simulink model "sampled_data_system"  (R2015a)
settings: Solver=ode45  StartTime=0.0  StopTime=tfinal  FixedStep=T  MaxStep=0.01  RelTol=1e-12  AbsTol=1e-12
values from neighbouring files (symbols this model uses):
  T = 0.004    [Fixed_Inner_Ctrl.mat]    (also in iop_control_design.m)
libraries: cstblocks x2
settings Model: CovHtmlReporting=off  Creator=cnielsen  LastModifiedBy=m4fisher
settings DataIOCC: LimitDataPoints=off  SignalLoggingSaveFormat=ModelDataLogs  SaveOutput=off  SaveTime=off  Refine=5
settings OptimizationCC: ExpressionDepthLimit=2147483647
settings DebuggingCC: UnderspecifiedInitializationDetection=Classic  MergeDetectMultiDrivingBlocksExec=none  SolverPrmCheckMsg=warning  FcnCallInpInsideContextMsg=EnableAllAsWarning  StateNameClashWarn=warning
settings GRTTargetCC: CombineOutputUpdateFcns=off  GRTInterface=on
settings ConfigurationSet: Description=Simscape Multibody

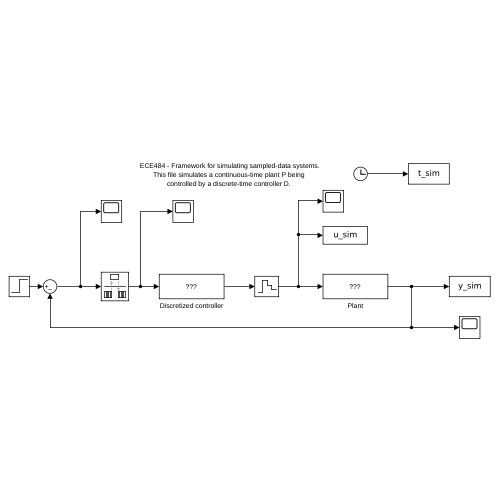
[thumbnail: Simulink's stored preview of the top-level diagram]
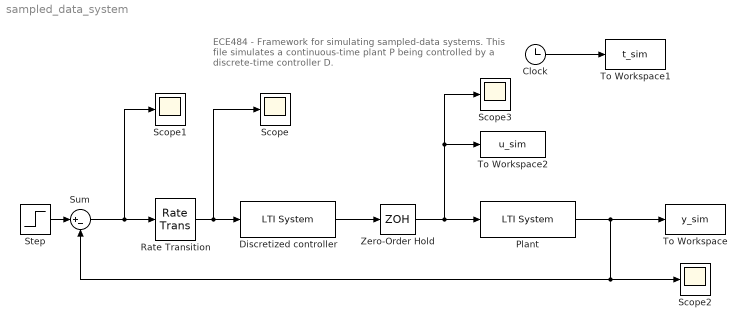
== system sampled_data_system ==
  note: ECE484 - Framework for simulating sampled-data systems.
      | This file simulates a continuous-time plant P being
      | controlled by a discrete-time controller D.
  Clock : Clock
  Discretized controller : cstblocks/LTI System  sys=D  IC=[]
  Plant : cstblocks/LTI System  sys=P  IC=[]
  Rate Transition : RateTransition  OutPortSampleTime=T
  Scope{,1..3} (4 alike) : Scope
      Scope settings: TimeRange=auto  MaxDataPoints=5000  SaveToWorkspace=off  YMin=-7.94103  YMax=8.76404  SampleTime=-1
      Scope1 settings: TimeRange=auto  MaxDataPoints=5000  SaveToWorkspace=off  YMin=-7.94103  YMax=8.76404  SampleTime=-1
      Scope2 settings: TimeRange=auto  MaxDataPoints=5000  SaveToWorkspace=off  SaveName=ScopeData2  YMin=-7.76404  YMax=8.94103  SampleTime=-1
      Scope3 settings: TimeRange=auto  MaxDataPoints=5000  SaveToWorkspace=off  SaveName=ScopeData  YMin=-15.91123  YMax=20.79205  SampleTime=-1
  Step : Step  Time=0
  Sum : Sum  Inputs=|+-
  To Workspace : ToWorkspace  VariableName=y_sim  SampleTime=-1
  To Workspace1 : ToWorkspace  VariableName=t_sim  SampleTime=-1
  To Workspace2 : ToWorkspace  VariableName=u_sim
  Zero-Order Hold : ZeroOrderHold  SampleTime=T
  wires:
  Clock/1 -> To Workspace1/1
  Discretized controller/1 -> Zero-Order Hold/1
  Step/1 -> Sum/1
  Plant/1 -> To Workspace/1, Sum/2, Scope2/1
  Sum/1 -> Rate Transition/1, Scope1/1
  Zero-Order Hold/1 -> Plant/1, To Workspace2/1, Scope3/1
  Rate Transition/1 -> Discretized controller/1, Scope/1
